simulink model "test1"  (R2019a)
settings: Solver=VariableStepAuto  StartTime=0.0  StopTime=10  RelTol=1e-3
settings Model: Creator=dell  LastModifiedBy=dell

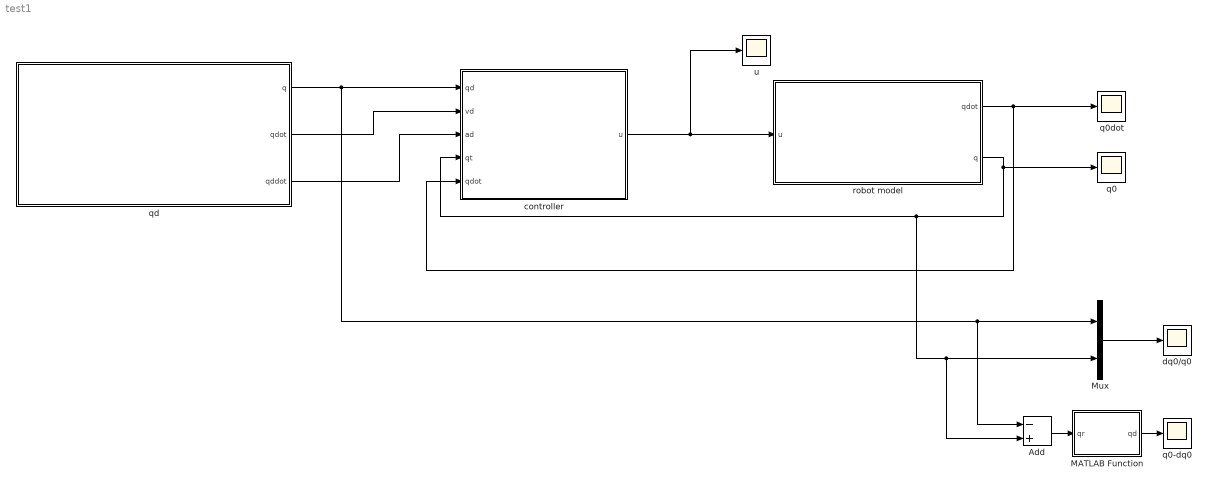
== system test1 ==
  Add : Sum  Inputs=-+
  MATLAB Function : MATLAB Function  TreatAsAtomicUnit=on
  Mux : Mux  Inputs=2
  controller : Subsystem
  dq0/q0 : Scope
  q0 : Scope
  q0-dq0 : Scope
  q0dot : Scope
  qd : Subsystem
  robot model : Subsystem
  u : Scope
  wires:
  qd/1(q) -> Add/1, Mux/1, controller/1(qd)
  qd/2(qdot) -> controller/2(vd)
  qd/3(qddot) -> controller/3(ad)
  robot model/2("q ") -> Add/2, Mux/2, controller/4(qt), q0/1
  robot model/1(qdot) -> q0dot/1, controller/5(qdot)
  Mux/1 -> dq0/q0/1
  Add/1 -> MATLAB Function/1(qr)
  MATLAB Function/1(qd) -> q0-dq0/1
  controller/1("u ") -> u/1, robot model/1(u)

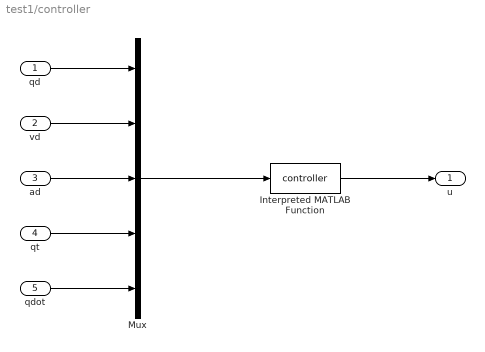
== system test1/controller ==
  qd : Inport
  vd : Inport  Port=2
  ad : Inport  Port=3
  qt : Inport  Port=4
  qdot : Inport  Port=5
  Interpreted MATLAB Function : MATLABFcn  MATLABFcn=controller
  Mux : Mux  Inputs=5
  "u " : Outport
  wires:
  Mux/1 -> Interpreted MATLAB Function/1
  qd/1 -> Mux/1
  Interpreted MATLAB Function/1 -> "u "/1
  vd/1 -> Mux/2
  ad/1 -> Mux/3
  qt/1 -> Mux/4
  qdot/1 -> Mux/5

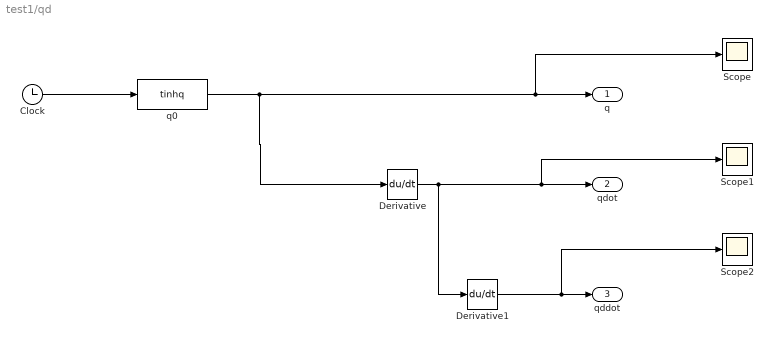
== system test1/qd ==
  Clock : Clock
      settings: Decimation=3
  Derivative : Derivative
  Derivative1 : Derivative
  Scope : Scope
  Scope1 : Scope
  Scope2 : Scope
  q0 : MATLABFcn  MATLABFcn=tinhq
  q : Outport
  qdot : Outport  Port=2
  qddot : Outport  Port=3
  wires:
  Clock/1 -> q0/1
  q0/1 -> q/1, Scope/1, Derivative/1
  Derivative/1 -> Derivative1/1, Scope1/1, qdot/1
  Derivative1/1 -> Scope2/1, qddot/1

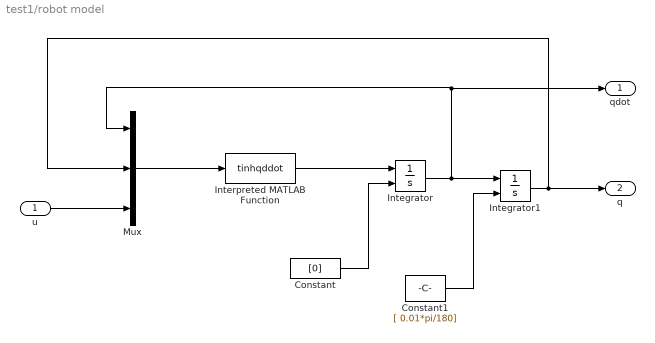
== system test1/robot model ==
  u : Inport
  Constant : Constant  Value=[0]
  Constant1 : Constant  Value=[ 0.01*pi/180]
  Integrator : Integrator  InitialConditionSource=external
  Integrator1 : Integrator  InitialConditionSource=external
  Interpreted MATLAB Function : MATLABFcn  MATLABFcn=tinhqddot
  Mux : Mux  Inputs=3
  qdot : Outport
  "q " : Outport  Port=2
  wires:
  Mux/1 -> Interpreted MATLAB Function/1
  Integrator/1 -> Mux/1, qdot/1, Integrator1/1
  u/1 -> Mux/3
  Integrator1/1 -> Mux/2, "q "/1
  Interpreted MATLAB Function/1 -> Integrator/1
  Constant/1 -> Integrator/2
  Constant1/1 -> Integrator1/2

== matlab function test1/MATLAB Function ==
  data: qr input; qd output
function qd = fcn(qr)
qd=qr*180/pi;
